simulink model "PROCESSSIMULATION"  (R2018b)
settings: Solver=VariableStepAuto  StartTime=0.0  StopTime=10  RelTol=1e-3
libraries: simulink_extras x7, powerlib x1
settings Model: Creator=Ratish Kumar S  LastModifiedBy=Ratish Kumar S

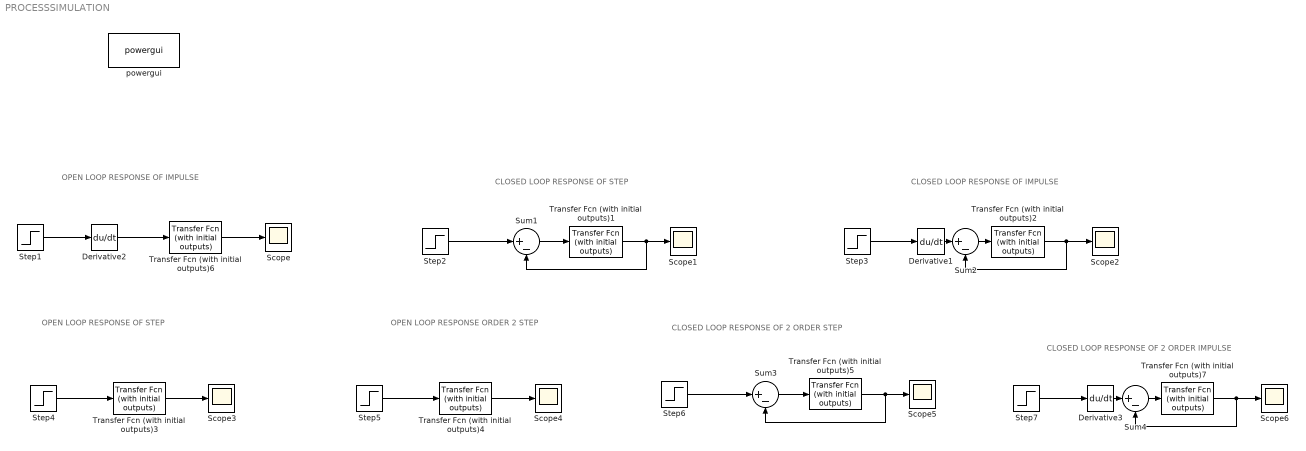
== system PROCESSSIMULATION ==
  note: CLOSED LOOP RESPONSE OF 2 ORDER IMPULSE
  note: CLOSED LOOP RESPONSE OF 2 ORDER STEP
  note: OPEN LOOP RESPONSE ORDER 2 STEP
  note: OPEN LOOP RESPONSE OF STEP
  note: OPEN LOOP RESPONSE OF IMPULSE
  note: CLOSED LOOP RESPONSE OF STEP
  note: CLOSED LOOP RESPONSE OF IMPULSE
  Derivative1 : Derivative
  Derivative2 : Derivative
  Derivative3 : Derivative
  Scope{,1..6} (7 alike) : Scope
  Step{1..7} (7 alike) : Step  Time=0  After=10  SampleTime=0
  Sum{1..4} (4 alike) : Sum  Inputs=|+-
  Transfer Fcn (with initial outputs){1..3,6} (4 alike) : simulink_extras/Additional Linear/Transfer Fcn (with initial outputs)  N=[4]  D="[1  2]"  Y0=.5  U0=0
  Transfer Fcn (with initial outputs)4 : simulink_extras/Additional Linear/Transfer Fcn (with initial outputs)  N=[4]  D=[ 1 6 16]  Y0=.5  U0=0
  Transfer Fcn (with initial outputs)5 : simulink_extras/Additional Linear/Transfer Fcn (with initial outputs)  N=[4]  D="[1  6 16]"  Y0=.5  U0=0
  Transfer Fcn (with initial outputs)7 : simulink_extras/Additional Linear/Transfer Fcn (with initial outputs)  N=[4]  D=[1 6 16]  Y0=.5  U0=0
  powergui : powerlib/powergui  Priority=1  SimulationMode=Continuous  SampleTime=50e-6  frequency=60  Iterations=50  frequencyindice=60  Pbase=100e6  ErrMax=1e-4  UnitsV=kV  UnitsW=MW  buscounter=0  FunctionMessages=off  echomessages=off  EnableUseOfTLC=off  CurrentSourceSwitches=off  DisableSnubberDevices=off  DisableRonSwitches=off  DisableVfSwitches=off  DisplayEquations=off  SolverType=Tustin/Backward Euler (TBE)  Interpol=off  ExternalGateDelay=off  methode=off  Ts=100  x0status=blocks  SPID=on  SwTol=0  HookPort=off  RestoreLinks=warning  ResistiveCurrentMeasurement=off  Frange=[0:2:500]  Ylog=off  Xlog=on  ShowGrid=off  save=off  variable=ZData  structure=0  ZoomFFT=off  StartTime=0.0  cycles=1  DisplayStyle=1  fundamental=60  FreqAxis=off  MaxFrequency=1000  frequencyindicesteady=1  RmsSteady=1  display=off
  wires:
  Step1/1 -> Derivative2/1
  Derivative2/1 -> Transfer Fcn (with initial outputs)6/1
  Transfer Fcn (with initial outputs)6/1 -> Scope/1
  Step2/1 -> Sum1/1
  Transfer Fcn (with initial outputs)1/1 -> Scope1/1, Sum1/2
  Sum1/1 -> Transfer Fcn (with initial outputs)1/1
  Transfer Fcn (with initial outputs)2/1 -> Sum2/2, Scope2/1
  Step3/1 -> Derivative1/1
  Derivative1/1 -> Sum2/1
  Sum2/1 -> Transfer Fcn (with initial outputs)2/1
  Step4/1 -> Transfer Fcn (with initial outputs)3/1
  Transfer Fcn (with initial outputs)3/1 -> Scope3/1
  Step5/1 -> Transfer Fcn (with initial outputs)4/1
  Transfer Fcn (with initial outputs)4/1 -> Scope4/1
  Sum3/1 -> Transfer Fcn (with initial outputs)5/1
  Step6/1 -> Sum3/1
  Transfer Fcn (with initial outputs)5/1 -> Scope5/1, Sum3/2
  Sum4/1 -> Transfer Fcn (with initial outputs)7/1
  Transfer Fcn (with initial outputs)7/1 -> Sum4/2, Scope6/1
  Step7/1 -> Derivative3/1
  Derivative3/1 -> Sum4/1
